simulink model "nn_12B"  (Simulink 10.0)
settings: Solver=ode45  StartTime=0  StopTime=100  RelTol=1e-3  EnableMultiTasking=on
values from neighbouring files (symbols this model uses):
  b1 = [-0.578256 -0.531049 0.449559 0.391358 0.277707 0.372638 -0.130073 0.423662 0.414256 -0.378106]    [nn_12B_data.mat]
  b2 = [-0.561938 -0.812212 -0.549473 -0.549797 -1.080223 0.652062 0.234581 1.306192 2.051893 -0.89138]    [nn_12B_data.mat]
  b3 = -0.01575    [nn_12B_data.mat]
  meaninp = [-0.014928 -0.08076]    [nn_12B_data.mat]
  meanout = -0.01416    [nn_12B_data.mat]
  oostdinp = [0.918012 0.847388]    [nn_12B_data.mat]
  stdevout = 0.183766    [nn_12B_data.mat]
  w1 = [-0.65101 1.000785 -0.225403 -1.250849 0.006928 0.402083 -0.27538 -0.375693 -0.343296 -0.963722 0.413488 0.166138 ... (20 elements, 2x10)]    [nn_12B_data.mat]
  w2 = [-0.059798 -0.128454 -0.107191 0.724165 -0.291639 -0.929753 -0.379182 0.996259 -0.416213 0.884865 -0.710416 -0.421403 ... (100 elements, 10x10)]    [nn_12B_data.mat]
  w3 = [-0.482061 0.739126 0.886125 1.875287 -0.959398 1.77256 -0.303801 0.909694 -0.681003 -0.930787]    [nn_12B_data.mat]
  xinmax = [1.885733 1.974943]    [nn_12B_data.mat]
  xinmin = [-1.969179 -1.999644]    [nn_12B_data.mat]
(part 1 of 2)
settings Model: Creator=niestma  LastModifiedBy=hbourbou
settings DataIOCC: LimitDataPoints=on
settings OptimizationCC: ExpressionDepthLimit=2147483647  LifeSpan=1  EfficientTunableParamExpr=on
settings DebuggingCC: StateNameClashWarn=warning
settings SFSimCC: MATLABDynamicMemAlloc=off
settings RTWCC: Description=Embedded Coder  SystemTargetFile=ert.tlc  TemplateMakefile=ert_default_tmf  GenerateReport=on  IncludeHyperlinkInReport=on  LaunchReport=on
settings CodeAppCC: IgnoreCustomStorageClasses=off  CustomSymbolStrType=$N$R$M  InternalIdentifier=Classic
settings ERTTargetCC: MultiwordLength=2048  GenerateSampleERTMain=on  ERTCustomFileTemplate=example_file_process.tlc  ConvertIfToSwitch=off  SuppressUnreachableDefaultCases=off
settings ConfigComp: CovExternalEMLEnable=off

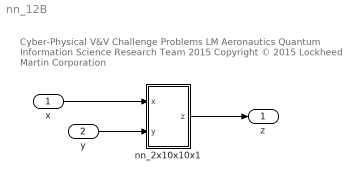
== system nn_12B ==
  note: Cyber-Physical V&V Challenge Problems
      | LM Aeronautics Quantum Information Science Research Team 2015
      | Copyright © 2015 Lockheed Martin Corporation
  x : Inport  OutDataTypeStr=double
  y : Inport  Port=2  OutDataTypeStr=double
  nn_2x10x10x1 : Subsystem
  z : Outport  VectorParamsAs1DForOutWhenUnconnected=off
  wires:
  nn_2x10x10x1/1(z) -> z/1
  x/1 -> nn_2x10x10x1/1(x)
  y/1 -> nn_2x10x10x1/2(y)

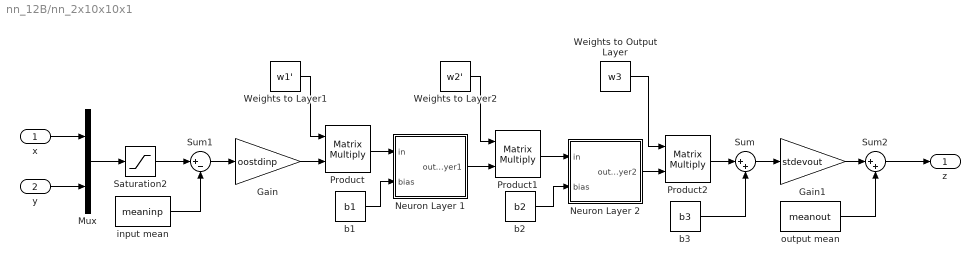
== system nn_12B/nn_2x10x10x1 ==
  x : Inport
  y : Inport  Port=2
  Gain : Gain  Gain=oostdinp
  Gain1 : Gain  Gain=stdevout
  Mux : Mux  Inputs=2
  Neuron Layer 1 : Subsystem
  Neuron Layer 2 : Subsystem
  Product : Product  Multiplication=Matrix(*)  RndMeth=Zero
  Product1 : Product  Multiplication=Matrix(*)  RndMeth=Zero
  Product2 : Product  Multiplication=Matrix(*)  RndMeth=Zero
  Saturation2 : Saturate  UpperLimit=xinmax  LowerLimit=xinmin
  Sum : Sum  Inputs=|++
  Sum1 : Sum  Inputs=|+-
  Sum2 : Sum  Inputs=|++
  Weights to Layer1 : Constant  Value=w1'  VectorParams1D=off
  Weights to Layer2 : Constant  Value=w2'  VectorParams1D=off
  Weights to Output Layer : Constant  Value=w3  VectorParams1D=off
  b1 : Constant  Value=b1
  b2 : Constant  Value=b2
  b3 : Constant  Value=b3
  input mean : Constant  Value=meaninp
  output mean : Constant  Value=meanout
  z : Outport  VectorParamsAs1DForOutWhenUnconnected=off
  wires:
  Product1/1 -> Neuron Layer 2/1(in)
  b2/1 -> Neuron Layer 2/2(bias)
  x/1 -> Mux/1
  b1/1 -> Neuron Layer 1/2(bias)
  b3/1 -> Sum/2
  y/1 -> Mux/2
  Weights to Layer1/1 -> Product/1
  Weights to Layer2/1 -> Product1/1
  Product/1 -> Neuron Layer 1/1(in)
  Neuron Layer 1/1(output layer1) -> Product1/2
  Weights to Output Layer/1 -> Product2/1
  Neuron Layer 2/1(output layer2) -> Product2/2
  Product2/1 -> Sum/1
  Mux/1 -> Saturation2/1
  Saturation2/1 -> Sum1/1
  input mean/1 -> Sum1/2
  Gain/1 -> Product/2
  Sum1/1 -> Gain/1
  Sum/1 -> Gain1/1
  Gain1/1 -> Sum2/1
  Sum2/1 -> z/1
  output mean/1 -> Sum2/2

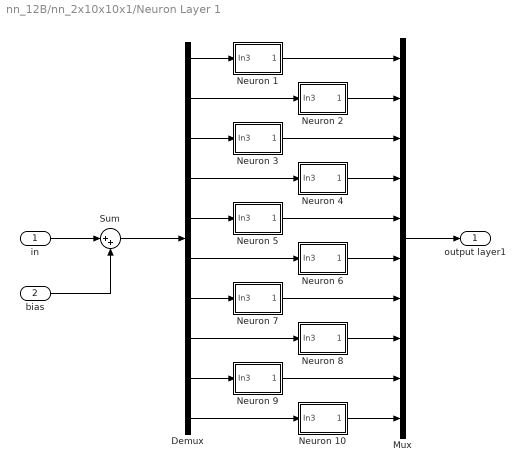
== system nn_12B/nn_2x10x10x1/Neuron Layer 1 ==
  in : Inport
  bias : Inport  Port=2
  Demux : Demux  Outputs=10
  Mux : Mux  Inputs=10
  Neuron 1 : Subsystem
  Neuron 10 : Subsystem
  Neuron 2 : Subsystem
  Neuron 3 : Subsystem
  Neuron 4 : Subsystem
  Neuron 5 : Subsystem
  Neuron 6 : Subsystem
  Neuron 7 : Subsystem
  Neuron 8 : Subsystem
  Neuron 9 : Subsystem
  Sum : Sum  Inputs=|++
  output layer1 : Outport  VectorParamsAs1DForOutWhenUnconnected=off
  wires:
  bias/1 -> Sum/2
  in/1 -> Sum/1
  Sum/1 -> Demux/1
  Demux/1 -> Neuron 1/1(In3)
  Neuron 1/1(Out1) -> Mux/1
  Mux/1 -> output layer1/1
  Neuron 2/1(Out1) -> Mux/2
  Demux/2 -> Neuron 2/1(In3)
  Demux/3 -> Neuron 3/1(In3)
  Neuron 3/1(Out1) -> Mux/3
  Demux/4 -> Neuron 4/1(In3)
  Neuron 4/1(Out1) -> Mux/4
  Demux/5 -> Neuron 5/1(In3)
  Neuron 5/1(Out1) -> Mux/5
  Demux/6 -> Neuron 6/1(In3)
  Demux/7 -> Neuron 7/1(In3)
  Neuron 7/1(Out1) -> Mux/7
  Demux/8 -> Neuron 8/1(In3)
  Neuron 6/1(Out1) -> Mux/6
  Neuron 8/1(Out1) -> Mux/8
  Demux/9 -> Neuron 9/1(In3)
  Neuron 9/1(Out1) -> Mux/9
  Demux/10 -> Neuron 10/1(In3)
  Neuron 10/1(Out1) -> Mux/10

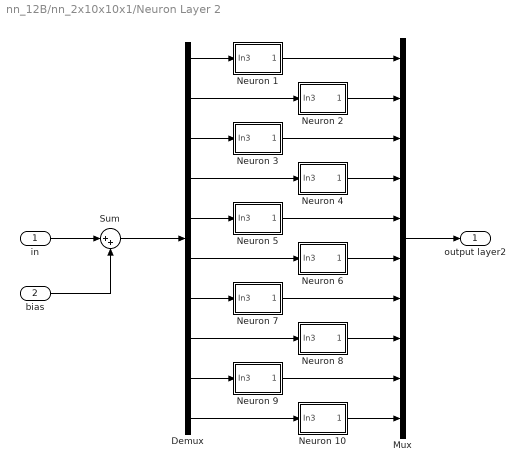
== system nn_12B/nn_2x10x10x1/Neuron Layer 2 ==
  in : Inport
  bias : Inport  Port=2
  Demux : Demux  Outputs=10
  Mux : Mux  Inputs=10
  Neuron 1 : Subsystem
  Neuron 10 : Subsystem
  Neuron 2 : Subsystem
  Neuron 3 : Subsystem
  Neuron 4 : Subsystem
  Neuron 5 : Subsystem
  Neuron 6 : Subsystem
  Neuron 7 : Subsystem
  Neuron 8 : Subsystem
  Neuron 9 : Subsystem
  Sum : Sum  Inputs=|++
  output layer2 : Outport  VectorParamsAs1DForOutWhenUnconnected=off
  wires:
  bias/1 -> Sum/2
  in/1 -> Sum/1
  Sum/1 -> Demux/1
  Demux/1 -> Neuron 1/1(In3)
  Neuron 1/1(Out1) -> Mux/1
  Mux/1 -> output layer2/1
  Neuron 2/1(Out1) -> Mux/2
  Demux/2 -> Neuron 2/1(In3)
  Demux/3 -> Neuron 3/1(In3)
  Neuron 3/1(Out1) -> Mux/3
  Demux/4 -> Neuron 4/1(In3)
  Neuron 4/1(Out1) -> Mux/4
  Demux/5 -> Neuron 5/1(In3)
  Neuron 5/1(Out1) -> Mux/5
  Demux/6 -> Neuron 6/1(In3)
  Demux/7 -> Neuron 7/1(In3)
  Neuron 7/1(Out1) -> Mux/7
  Demux/8 -> Neuron 8/1(In3)
  Neuron 6/1(Out1) -> Mux/6
  Neuron 8/1(Out1) -> Mux/8
  Demux/9 -> Neuron 9/1(In3)
  Neuron 9/1(Out1) -> Mux/9
  Demux/10 -> Neuron 10/1(In3)
  Neuron 10/1(Out1) -> Mux/10

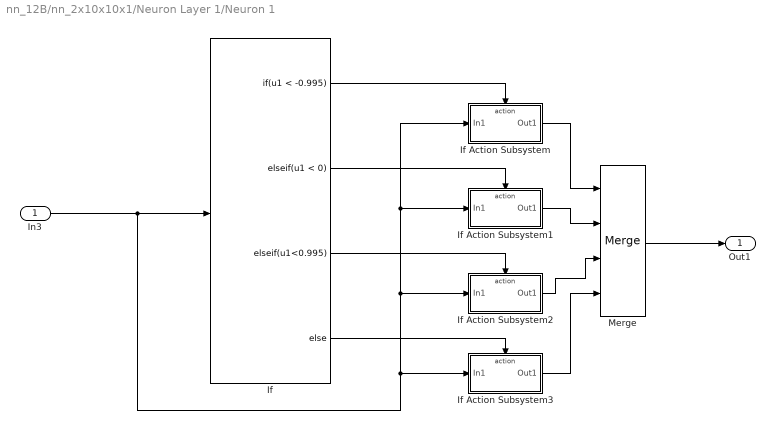
== system nn_12B/nn_2x10x10x1/Neuron Layer 1/Neuron 1 ==
  In3 : Inport
  If : If  IfExpression=u1 < -0.995  ElseIfExpressions=u1 < 0, u1<0.995
  If Action Subsystem : Subsystem  TreatAsAtomicUnit=on
  If Action Subsystem1 : Subsystem  TreatAsAtomicUnit=on
  If Action Subsystem2 : Subsystem  TreatAsAtomicUnit=on
  If Action Subsystem3 : Subsystem  TreatAsAtomicUnit=on
  Merge : Merge  Inputs=4
  Out1 : Outport  VectorParamsAs1DForOutWhenUnconnected=off
  wires:
  If/1 -> If Action Subsystem/Action
  If/2 -> If Action Subsystem1/Action
  If/3 -> If Action Subsystem2/Action
  If/4 -> If Action Subsystem3/Action
  If Action Subsystem/1(Out1) -> Merge/1
  If Action Subsystem3/1(Out1) -> Merge/4
  If Action Subsystem1/1(Out1) -> Merge/2
  If Action Subsystem2/1(Out1) -> Merge/3
  In3/1 -> If Action Subsystem3/1(In1), If Action Subsystem2/1(In1), If Action Subsystem1/1(In1), If Action Subsystem/1(In1), If/1
  Merge/1 -> Out1/1

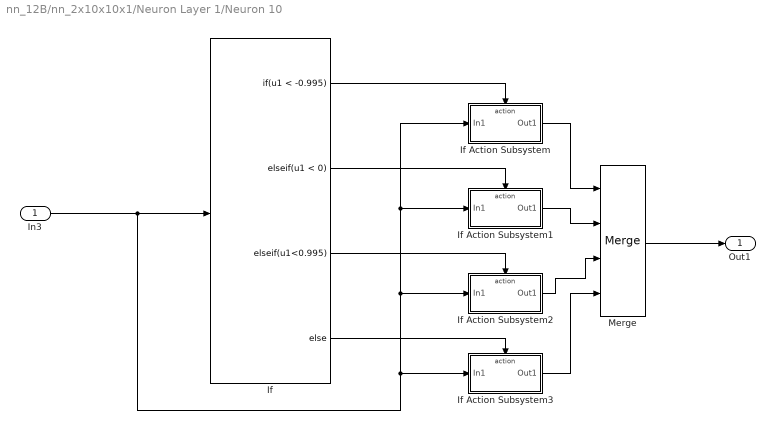
== system nn_12B/nn_2x10x10x1/Neuron Layer 1/Neuron 10 ==
  In3 : Inport
  If : If  IfExpression=u1 < -0.995  ElseIfExpressions=u1 < 0, u1<0.995
  If Action Subsystem : Subsystem  TreatAsAtomicUnit=on
  If Action Subsystem1 : Subsystem  TreatAsAtomicUnit=on
  If Action Subsystem2 : Subsystem  TreatAsAtomicUnit=on
  If Action Subsystem3 : Subsystem  TreatAsAtomicUnit=on
  Merge : Merge  Inputs=4
  Out1 : Outport  VectorParamsAs1DForOutWhenUnconnected=off
  wires:
  Merge/1 -> Out1/1
  In3/1 -> If/1, If Action Subsystem/1(In1), If Action Subsystem1/1(In1), If Action Subsystem2/1(In1), If Action Subsystem3/1(In1)
  If Action Subsystem2/1(Out1) -> Merge/3
  If Action Subsystem1/1(Out1) -> Merge/2
  If Action Subsystem3/1(Out1) -> Merge/4
  If Action Subsystem/1(Out1) -> Merge/1
  If/4 -> If Action Subsystem3/Action
  If/3 -> If Action Subsystem2/Action
  If/2 -> If Action Subsystem1/Action
  If/1 -> If Action Subsystem/Action

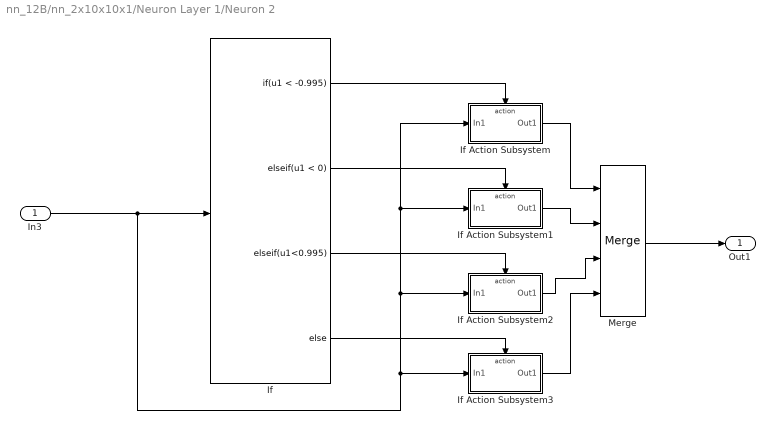
== system nn_12B/nn_2x10x10x1/Neuron Layer 1/Neuron 2 ==
  In3 : Inport
  If : If  IfExpression=u1 < -0.995  ElseIfExpressions=u1 < 0, u1<0.995
  If Action Subsystem : Subsystem  TreatAsAtomicUnit=on
  If Action Subsystem1 : Subsystem  TreatAsAtomicUnit=on
  If Action Subsystem2 : Subsystem  TreatAsAtomicUnit=on
  If Action Subsystem3 : Subsystem  TreatAsAtomicUnit=on
  Merge : Merge  Inputs=4
  Out1 : Outport  VectorParamsAs1DForOutWhenUnconnected=off
  wires:
  Merge/1 -> Out1/1
  In3/1 -> If/1, If Action Subsystem/1(In1), If Action Subsystem1/1(In1), If Action Subsystem2/1(In1), If Action Subsystem3/1(In1)
  If Action Subsystem2/1(Out1) -> Merge/3
  If Action Subsystem1/1(Out1) -> Merge/2
  If Action Subsystem3/1(Out1) -> Merge/4
  If Action Subsystem/1(Out1) -> Merge/1
  If/4 -> If Action Subsystem3/Action
  If/3 -> If Action Subsystem2/Action
  If/2 -> If Action Subsystem1/Action
  If/1 -> If Action Subsystem/Action

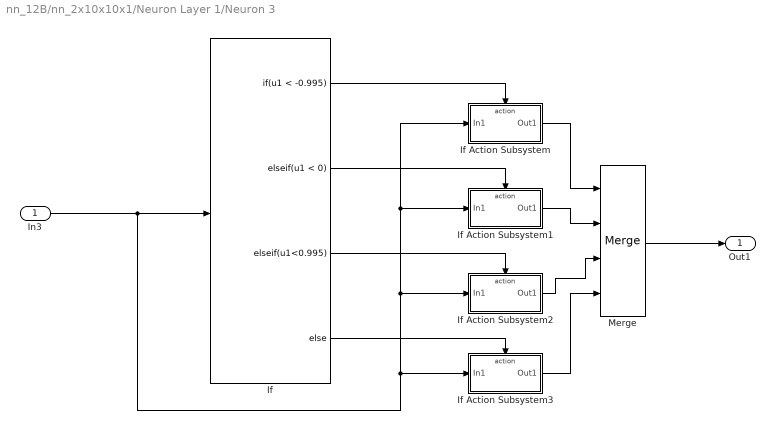
== system nn_12B/nn_2x10x10x1/Neuron Layer 1/Neuron 3 ==
  In3 : Inport
  If : If  IfExpression=u1 < -0.995  ElseIfExpressions=u1 < 0, u1<0.995
  If Action Subsystem : Subsystem  TreatAsAtomicUnit=on
  If Action Subsystem1 : Subsystem  TreatAsAtomicUnit=on
  If Action Subsystem2 : Subsystem  TreatAsAtomicUnit=on
  If Action Subsystem3 : Subsystem  TreatAsAtomicUnit=on
  Merge : Merge  Inputs=4
  Out1 : Outport  VectorParamsAs1DForOutWhenUnconnected=off
  wires:
  If/1 -> If Action Subsystem/Action
  If/2 -> If Action Subsystem1/Action
  If/3 -> If Action Subsystem2/Action
  If/4 -> If Action Subsystem3/Action
  If Action Subsystem/1(Out1) -> Merge/1
  If Action Subsystem3/1(Out1) -> Merge/4
  If Action Subsystem1/1(Out1) -> Merge/2
  If Action Subsystem2/1(Out1) -> Merge/3
  In3/1 -> If Action Subsystem3/1(In1), If Action Subsystem2/1(In1), If Action Subsystem1/1(In1), If Action Subsystem/1(In1), If/1
  Merge/1 -> Out1/1

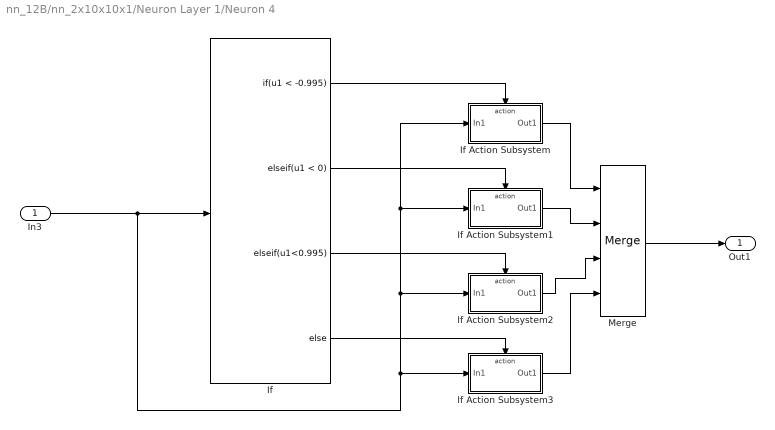
== system nn_12B/nn_2x10x10x1/Neuron Layer 1/Neuron 4 ==
  In3 : Inport
  If : If  IfExpression=u1 < -0.995  ElseIfExpressions=u1 < 0, u1<0.995
  If Action Subsystem : Subsystem  TreatAsAtomicUnit=on
  If Action Subsystem1 : Subsystem  TreatAsAtomicUnit=on
  If Action Subsystem2 : Subsystem  TreatAsAtomicUnit=on
  If Action Subsystem3 : Subsystem  TreatAsAtomicUnit=on
  Merge : Merge  Inputs=4
  Out1 : Outport  VectorParamsAs1DForOutWhenUnconnected=off
  wires:
  If/1 -> If Action Subsystem/Action
  If/2 -> If Action Subsystem1/Action
  If/3 -> If Action Subsystem2/Action
  If/4 -> If Action Subsystem3/Action
  If Action Subsystem/1(Out1) -> Merge/1
  If Action Subsystem3/1(Out1) -> Merge/4
  If Action Subsystem1/1(Out1) -> Merge/2
  If Action Subsystem2/1(Out1) -> Merge/3
  In3/1 -> If Action Subsystem3/1(In1), If Action Subsystem2/1(In1), If Action Subsystem1/1(In1), If Action Subsystem/1(In1), If/1
  Merge/1 -> Out1/1

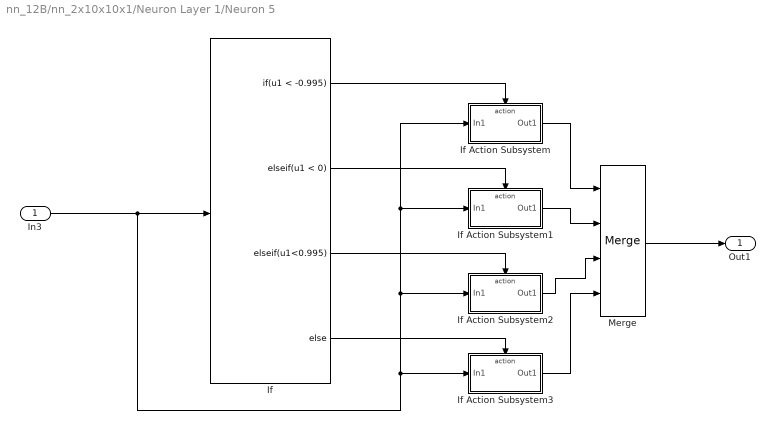
== system nn_12B/nn_2x10x10x1/Neuron Layer 1/Neuron 5 ==
  In3 : Inport
  If : If  IfExpression=u1 < -0.995  ElseIfExpressions=u1 < 0, u1<0.995
  If Action Subsystem : Subsystem  TreatAsAtomicUnit=on
  If Action Subsystem1 : Subsystem  TreatAsAtomicUnit=on
  If Action Subsystem2 : Subsystem  TreatAsAtomicUnit=on
  If Action Subsystem3 : Subsystem  TreatAsAtomicUnit=on
  Merge : Merge  Inputs=4
  Out1 : Outport  VectorParamsAs1DForOutWhenUnconnected=off
  wires:
  If/1 -> If Action Subsystem/Action
  If/2 -> If Action Subsystem1/Action
  If/3 -> If Action Subsystem2/Action
  If/4 -> If Action Subsystem3/Action
  If Action Subsystem/1(Out1) -> Merge/1
  If Action Subsystem3/1(Out1) -> Merge/4
  If Action Subsystem1/1(Out1) -> Merge/2
  If Action Subsystem2/1(Out1) -> Merge/3
  In3/1 -> If Action Subsystem3/1(In1), If Action Subsystem2/1(In1), If Action Subsystem1/1(In1), If Action Subsystem/1(In1), If/1
  Merge/1 -> Out1/1

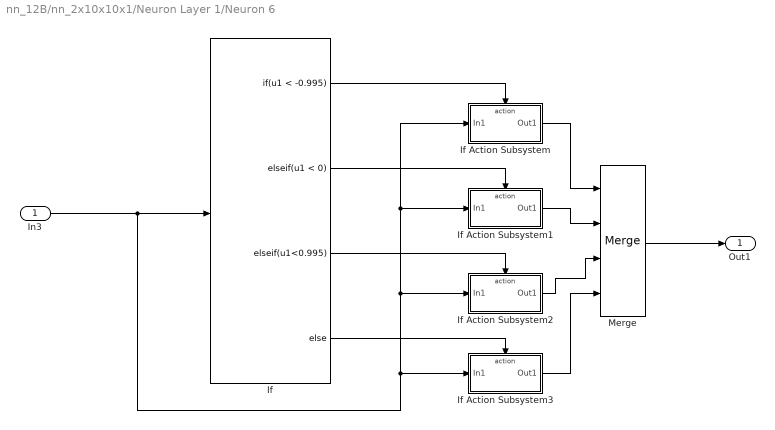
== system nn_12B/nn_2x10x10x1/Neuron Layer 1/Neuron 6 ==
  In3 : Inport
  If : If  IfExpression=u1 < -0.995  ElseIfExpressions=u1 < 0, u1<0.995
  If Action Subsystem : Subsystem  TreatAsAtomicUnit=on
  If Action Subsystem1 : Subsystem  TreatAsAtomicUnit=on
  If Action Subsystem2 : Subsystem  TreatAsAtomicUnit=on
  If Action Subsystem3 : Subsystem  TreatAsAtomicUnit=on
  Merge : Merge  Inputs=4
  Out1 : Outport  VectorParamsAs1DForOutWhenUnconnected=off
  wires:
  Merge/1 -> Out1/1
  In3/1 -> If/1, If Action Subsystem/1(In1), If Action Subsystem1/1(In1), If Action Subsystem2/1(In1), If Action Subsystem3/1(In1)
  If Action Subsystem2/1(Out1) -> Merge/3
  If Action Subsystem1/1(Out1) -> Merge/2
  If Action Subsystem3/1(Out1) -> Merge/4
  If Action Subsystem/1(Out1) -> Merge/1
  If/4 -> If Action Subsystem3/Action
  If/3 -> If Action Subsystem2/Action
  If/2 -> If Action Subsystem1/Action
  If/1 -> If Action Subsystem/Action

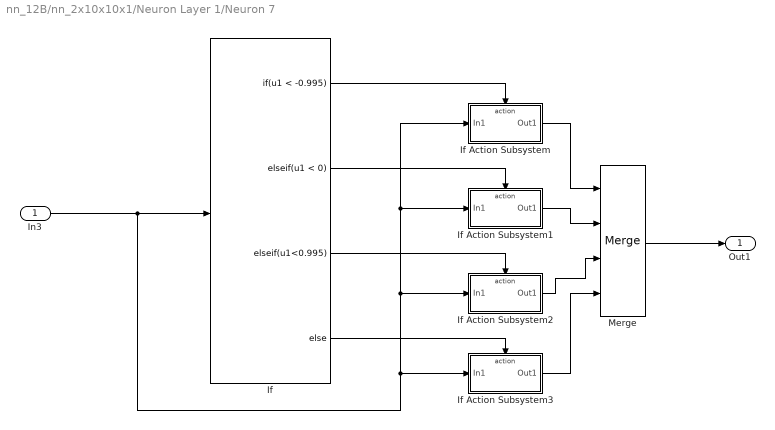
== system nn_12B/nn_2x10x10x1/Neuron Layer 1/Neuron 7 ==
  In3 : Inport
  If : If  IfExpression=u1 < -0.995  ElseIfExpressions=u1 < 0, u1<0.995
  If Action Subsystem : Subsystem  TreatAsAtomicUnit=on
  If Action Subsystem1 : Subsystem  TreatAsAtomicUnit=on
  If Action Subsystem2 : Subsystem  TreatAsAtomicUnit=on
  If Action Subsystem3 : Subsystem  TreatAsAtomicUnit=on
  Merge : Merge  Inputs=4
  Out1 : Outport  VectorParamsAs1DForOutWhenUnconnected=off
  wires:
  If/1 -> If Action Subsystem/Action
  If/2 -> If Action Subsystem1/Action
  If/3 -> If Action Subsystem2/Action
  If/4 -> If Action Subsystem3/Action
  If Action Subsystem/1(Out1) -> Merge/1
  If Action Subsystem3/1(Out1) -> Merge/4
  If Action Subsystem1/1(Out1) -> Merge/2
  If Action Subsystem2/1(Out1) -> Merge/3
  In3/1 -> If Action Subsystem3/1(In1), If Action Subsystem2/1(In1), If Action Subsystem1/1(In1), If Action Subsystem/1(In1), If/1
  Merge/1 -> Out1/1

== system nn_12B/nn_2x10x10x1/Neuron Layer 1/Neuron 8 ==
  In3 : Inport
  If : If  IfExpression=u1 < -0.995  ElseIfExpressions=u1 < 0, u1<0.995
  If Action Subsystem : Subsystem  TreatAsAtomicUnit=on
  If Action Subsystem1 : Subsystem  TreatAsAtomicUnit=on
  If Action Subsystem2 : Subsystem  TreatAsAtomicUnit=on
  If Action Subsystem3 : Subsystem  TreatAsAtomicUnit=on
  Merge : Merge  Inputs=4
  Out1 : Outport  VectorParamsAs1DForOutWhenUnconnected=off
  wires:
  If/1 -> If Action Subsystem/Action
  If/2 -> If Action Subsystem1/Action
  If/3 -> If Action Subsystem2/Action
  If/4 -> If Action Subsystem3/Action
  If Action Subsystem/1(Out1) -> Merge/1
  If Action Subsystem3/1(Out1) -> Merge/4
  If Action Subsystem1/1(Out1) -> Merge/2
  If Action Subsystem2/1(Out1) -> Merge/3
  In3/1 -> If Action Subsystem3/1(In1), If Action Subsystem2/1(In1), If Action Subsystem1/1(In1), If Action Subsystem/1(In1), If/1
  Merge/1 -> Out1/1

== system nn_12B/nn_2x10x10x1/Neuron Layer 1/Neuron 9 ==
  In3 : Inport
  If : If  IfExpression=u1 < -0.995  ElseIfExpressions=u1 < 0, u1<0.995
  If Action Subsystem : Subsystem  TreatAsAtomicUnit=on
  If Action Subsystem1 : Subsystem  TreatAsAtomicUnit=on
  If Action Subsystem2 : Subsystem  TreatAsAtomicUnit=on
  If Action Subsystem3 : Subsystem  TreatAsAtomicUnit=on
  Merge : Merge  Inputs=4
  Out1 : Outport  VectorParamsAs1DForOutWhenUnconnected=off
  wires:
  If/1 -> If Action Subsystem/Action
  If/2 -> If Action Subsystem1/Action
  If/3 -> If Action Subsystem2/Action
  If/4 -> If Action Subsystem3/Action
  If Action Subsystem/1(Out1) -> Merge/1
  If Action Subsystem3/1(Out1) -> Merge/4
  If Action Subsystem1/1(Out1) -> Merge/2
  If Action Subsystem2/1(Out1) -> Merge/3
  In3/1 -> If Action Subsystem3/1(In1), If Action Subsystem2/1(In1), If Action Subsystem1/1(In1), If Action Subsystem/1(In1), If/1
  Merge/1 -> Out1/1

== system nn_12B/nn_2x10x10x1/Neuron Layer 2/Neuron 1 ==
  In3 : Inport
  If : If  IfExpression=u1 < -0.995  ElseIfExpressions=u1 < 0, u1<0.995
  If Action Subsystem : Subsystem  TreatAsAtomicUnit=on
  If Action Subsystem1 : Subsystem  TreatAsAtomicUnit=on
  If Action Subsystem2 : Subsystem  TreatAsAtomicUnit=on
  If Action Subsystem3 : Subsystem  TreatAsAtomicUnit=on
  Merge : Merge  Inputs=4
  Out1 : Outport  VectorParamsAs1DForOutWhenUnconnected=off
  wires:
  If/1 -> If Action Subsystem/Action
  If/2 -> If Action Subsystem1/Action
  If/3 -> If Action Subsystem2/Action
  If/4 -> If Action Subsystem3/Action
  If Action Subsystem/1(Out1) -> Merge/1
  If Action Subsystem3/1(Out1) -> Merge/4
  If Action Subsystem1/1(Out1) -> Merge/2
  If Action Subsystem2/1(Out1) -> Merge/3
  In3/1 -> If Action Subsystem3/1(In1), If Action Subsystem2/1(In1), If Action Subsystem1/1(In1), If Action Subsystem/1(In1), If/1
  Merge/1 -> Out1/1

== system nn_12B/nn_2x10x10x1/Neuron Layer 2/Neuron 10 ==
  In3 : Inport
  If : If  IfExpression=u1 < -0.995  ElseIfExpressions=u1 < 0, u1<0.995
  If Action Subsystem : Subsystem  TreatAsAtomicUnit=on
  If Action Subsystem1 : Subsystem  TreatAsAtomicUnit=on
  If Action Subsystem2 : Subsystem  TreatAsAtomicUnit=on
  If Action Subsystem3 : Subsystem  TreatAsAtomicUnit=on
  Merge : Merge  Inputs=4
  Out1 : Outport  VectorParamsAs1DForOutWhenUnconnected=off
  wires:
  Merge/1 -> Out1/1
  In3/1 -> If/1, If Action Subsystem/1(In1), If Action Subsystem1/1(In1), If Action Subsystem2/1(In1), If Action Subsystem3/1(In1)
  If Action Subsystem2/1(Out1) -> Merge/3
  If Action Subsystem1/1(Out1) -> Merge/2
  If Action Subsystem3/1(Out1) -> Merge/4
  If Action Subsystem/1(Out1) -> Merge/1
  If/4 -> If Action Subsystem3/Action
  If/3 -> If Action Subsystem2/Action
  If/2 -> If Action Subsystem1/Action
  If/1 -> If Action Subsystem/Action

== system nn_12B/nn_2x10x10x1/Neuron Layer 2/Neuron 2 ==
  In3 : Inport
  If : If  IfExpression=u1 < -0.995  ElseIfExpressions=u1 < 0, u1<0.995
  If Action Subsystem : Subsystem  TreatAsAtomicUnit=on
  If Action Subsystem1 : Subsystem  TreatAsAtomicUnit=on
  If Action Subsystem2 : Subsystem  TreatAsAtomicUnit=on
  If Action Subsystem3 : Subsystem  TreatAsAtomicUnit=on
  Merge : Merge  Inputs=4
  Out1 : Outport  VectorParamsAs1DForOutWhenUnconnected=off
  wires:
  Merge/1 -> Out1/1
  In3/1 -> If/1, If Action Subsystem/1(In1), If Action Subsystem1/1(In1), If Action Subsystem2/1(In1), If Action Subsystem3/1(In1)
  If Action Subsystem2/1(Out1) -> Merge/3
  If Action Subsystem1/1(Out1) -> Merge/2
  If Action Subsystem3/1(Out1) -> Merge/4
  If Action Subsystem/1(Out1) -> Merge/1
  If/4 -> If Action Subsystem3/Action
  If/3 -> If Action Subsystem2/Action
  If/2 -> If Action Subsystem1/Action
  If/1 -> If Action Subsystem/Action

== system nn_12B/nn_2x10x10x1/Neuron Layer 2/Neuron 3 ==
  In3 : Inport
  If : If  IfExpression=u1 < -0.995  ElseIfExpressions=u1 < 0, u1<0.995
  If Action Subsystem : Subsystem  TreatAsAtomicUnit=on
  If Action Subsystem1 : Subsystem  TreatAsAtomicUnit=on
  If Action Subsystem2 : Subsystem  TreatAsAtomicUnit=on
  If Action Subsystem3 : Subsystem  TreatAsAtomicUnit=on
  Merge : Merge  Inputs=4
  Out1 : Outport  VectorParamsAs1DForOutWhenUnconnected=off
  wires:
  If/1 -> If Action Subsystem/Action
  If/2 -> If Action Subsystem1/Action
  If/3 -> If Action Subsystem2/Action
  If/4 -> If Action Subsystem3/Action
  If Action Subsystem/1(Out1) -> Merge/1
  If Action Subsystem3/1(Out1) -> Merge/4
  If Action Subsystem1/1(Out1) -> Merge/2
  If Action Subsystem2/1(Out1) -> Merge/3
  In3/1 -> If Action Subsystem3/1(In1), If Action Subsystem2/1(In1), If Action Subsystem1/1(In1), If Action Subsystem/1(In1), If/1
  Merge/1 -> Out1/1

== system nn_12B/nn_2x10x10x1/Neuron Layer 2/Neuron 4 ==
  In3 : Inport
  If : If  IfExpression=u1 < -0.995  ElseIfExpressions=u1 < 0, u1<0.995
  If Action Subsystem : Subsystem  TreatAsAtomicUnit=on
  If Action Subsystem1 : Subsystem  TreatAsAtomicUnit=on
  If Action Subsystem2 : Subsystem  TreatAsAtomicUnit=on
  If Action Subsystem3 : Subsystem  TreatAsAtomicUnit=on
  Merge : Merge  Inputs=4
  Out1 : Outport  VectorParamsAs1DForOutWhenUnconnected=off
  wires:
  If/1 -> If Action Subsystem/Action
  If/2 -> If Action Subsystem1/Action
  If/3 -> If Action Subsystem2/Action
  If/4 -> If Action Subsystem3/Action
  If Action Subsystem/1(Out1) -> Merge/1
  If Action Subsystem3/1(Out1) -> Merge/4
  If Action Subsystem1/1(Out1) -> Merge/2
  If Action Subsystem2/1(Out1) -> Merge/3
  In3/1 -> If Action Subsystem3/1(In1), If Action Subsystem2/1(In1), If Action Subsystem1/1(In1), If Action Subsystem/1(In1), If/1
  Merge/1 -> Out1/1

== system nn_12B/nn_2x10x10x1/Neuron Layer 2/Neuron 5 ==
  In3 : Inport
  If : If  IfExpression=u1 < -0.995  ElseIfExpressions=u1 < 0, u1<0.995
  If Action Subsystem : Subsystem  TreatAsAtomicUnit=on
  If Action Subsystem1 : Subsystem  TreatAsAtomicUnit=on
  If Action Subsystem2 : Subsystem  TreatAsAtomicUnit=on
  If Action Subsystem3 : Subsystem  TreatAsAtomicUnit=on
  Merge : Merge  Inputs=4
  Out1 : Outport  VectorParamsAs1DForOutWhenUnconnected=off
  wires:
  If/1 -> If Action Subsystem/Action
  If/2 -> If Action Subsystem1/Action
  If/3 -> If Action Subsystem2/Action
  If/4 -> If Action Subsystem3/Action
  If Action Subsystem/1(Out1) -> Merge/1
  If Action Subsystem3/1(Out1) -> Merge/4
  If Action Subsystem1/1(Out1) -> Merge/2
  If Action Subsystem2/1(Out1) -> Merge/3
  In3/1 -> If Action Subsystem3/1(In1), If Action Subsystem2/1(In1), If Action Subsystem1/1(In1), If Action Subsystem/1(In1), If/1
  Merge/1 -> Out1/1

== system nn_12B/nn_2x10x10x1/Neuron Layer 2/Neuron 6 ==
  In3 : Inport
  If : If  IfExpression=u1 < -0.995  ElseIfExpressions=u1 < 0, u1<0.995
  If Action Subsystem : Subsystem  TreatAsAtomicUnit=on
  If Action Subsystem1 : Subsystem  TreatAsAtomicUnit=on
  If Action Subsystem2 : Subsystem  TreatAsAtomicUnit=on
  If Action Subsystem3 : Subsystem  TreatAsAtomicUnit=on
  Merge : Merge  Inputs=4
  Out1 : Outport  VectorParamsAs1DForOutWhenUnconnected=off
  wires:
  Merge/1 -> Out1/1
  In3/1 -> If/1, If Action Subsystem/1(In1), If Action Subsystem1/1(In1), If Action Subsystem2/1(In1), If Action Subsystem3/1(In1)
  If Action Subsystem2/1(Out1) -> Merge/3
  If Action Subsystem1/1(Out1) -> Merge/2
  If Action Subsystem3/1(Out1) -> Merge/4
  If Action Subsystem/1(Out1) -> Merge/1
  If/4 -> If Action Subsystem3/Action
  If/3 -> If Action Subsystem2/Action
  If/2 -> If Action Subsystem1/Action
  If/1 -> If Action Subsystem/Action

== system nn_12B/nn_2x10x10x1/Neuron Layer 2/Neuron 7 ==
  In3 : Inport
  If : If  IfExpression=u1 < -0.995  ElseIfExpressions=u1 < 0, u1<0.995
  If Action Subsystem : Subsystem  TreatAsAtomicUnit=on
  If Action Subsystem1 : Subsystem  TreatAsAtomicUnit=on
  If Action Subsystem2 : Subsystem  TreatAsAtomicUnit=on
  If Action Subsystem3 : Subsystem  TreatAsAtomicUnit=on
  Merge : Merge  Inputs=4
  Out1 : Outport  VectorParamsAs1DForOutWhenUnconnected=off
  wires:
  If/1 -> If Action Subsystem/Action
  If/2 -> If Action Subsystem1/Action
  If/3 -> If Action Subsystem2/Action
  If/4 -> If Action Subsystem3/Action
  If Action Subsystem/1(Out1) -> Merge/1
  If Action Subsystem3/1(Out1) -> Merge/4
  If Action Subsystem1/1(Out1) -> Merge/2
  If Action Subsystem2/1(Out1) -> Merge/3
  In3/1 -> If Action Subsystem3/1(In1), If Action Subsystem2/1(In1), If Action Subsystem1/1(In1), If Action Subsystem/1(In1), If/1
  Merge/1 -> Out1/1

== system nn_12B/nn_2x10x10x1/Neuron Layer 2/Neuron 8 ==
  In3 : Inport
  If : If  IfExpression=u1 < -0.995  ElseIfExpressions=u1 < 0, u1<0.995
  If Action Subsystem : Subsystem  TreatAsAtomicUnit=on
  If Action Subsystem1 : Subsystem  TreatAsAtomicUnit=on
  If Action Subsystem2 : Subsystem  TreatAsAtomicUnit=on
  If Action Subsystem3 : Subsystem  TreatAsAtomicUnit=on
  Merge : Merge  Inputs=4
  Out1 : Outport  VectorParamsAs1DForOutWhenUnconnected=off
  wires:
  If/1 -> If Action Subsystem/Action
  If/2 -> If Action Subsystem1/Action
  If/3 -> If Action Subsystem2/Action
  If/4 -> If Action Subsystem3/Action
  If Action Subsystem/1(Out1) -> Merge/1
  If Action Subsystem3/1(Out1) -> Merge/4
  If Action Subsystem1/1(Out1) -> Merge/2
  If Action Subsystem2/1(Out1) -> Merge/3
  In3/1 -> If Action Subsystem3/1(In1), If Action Subsystem2/1(In1), If Action Subsystem1/1(In1), If Action Subsystem/1(In1), If/1
  Merge/1 -> Out1/1

== system nn_12B/nn_2x10x10x1/Neuron Layer 2/Neuron 9 ==
  In3 : Inport
  If : If  IfExpression=u1 < -0.995  ElseIfExpressions=u1 < 0, u1<0.995
  If Action Subsystem : Subsystem  TreatAsAtomicUnit=on
  If Action Subsystem1 : Subsystem  TreatAsAtomicUnit=on
  If Action Subsystem2 : Subsystem  TreatAsAtomicUnit=on
  If Action Subsystem3 : Subsystem  TreatAsAtomicUnit=on
  Merge : Merge  Inputs=4
  Out1 : Outport  VectorParamsAs1DForOutWhenUnconnected=off
  wires:
  If/1 -> If Action Subsystem/Action
  If/2 -> If Action Subsystem1/Action
  If/3 -> If Action Subsystem2/Action
  If/4 -> If Action Subsystem3/Action
  If Action Subsystem/1(Out1) -> Merge/1
  If Action Subsystem3/1(Out1) -> Merge/4
  If Action Subsystem1/1(Out1) -> Merge/2
  If Action Subsystem2/1(Out1) -> Merge/3
  In3/1 -> If Action Subsystem3/1(In1), If Action Subsystem2/1(In1), If Action Subsystem1/1(In1), If Action Subsystem/1(In1), If/1
  Merge/1 -> Out1/1

== system nn_12B/nn_2x10x10x1/Neuron Layer 1/Neuron 1/If Action Subsystem ==
  In1 : Inport
  Action Port : ActionPort  ActionPortLabel=if { }
  Sum : Sum  Inputs=|+-
  bias1 : Constant  Value=0.990025
  weight1 : Gain  Gain=0.01
  Out1 : Outport  VectorParamsAs1DForOutWhenUnconnected=off
  wires:
  bias1/1 -> Sum/2
  weight1/1 -> Sum/1
  In1/1 -> weight1/1
  Sum/1 -> Out1/1

== system nn_12B/nn_2x10x10x1/Neuron Layer 1/Neuron 1/If Action Subsystem1 ==
  In1 : Inport
  Action Port : ActionPort  ActionPortLabel=elseif { }
  Product1 : Product  RndMeth=Zero
  Sum3 : Sum  Inputs=|++
  bias4 : Constant  Value=2
  Out1 : Outport  VectorParamsAs1DForOutWhenUnconnected=off
  wires:
  In1/1 -> Product1/1, Sum3/1
  bias4/1 -> Sum3/2
  Sum3/1 -> Product1/2
  Product1/1 -> Out1/1

== system nn_12B/nn_2x10x10x1/Neuron Layer 1/Neuron 1/If Action Subsystem2 ==
  In1 : Inport
  Action Port : ActionPort  ActionPortLabel=elseif { }
  Product1 : Product  RndMeth=Zero
  Sum3 : Sum  Inputs=|-+
  bias4 : Constant  Value=2
  Out1 : Outport  VectorParamsAs1DForOutWhenUnconnected=off
  wires:
  Product1/1 -> Out1/1
  Sum3/1 -> Product1/2
  bias4/1 -> Sum3/2
  In1/1 -> Sum3/1, Product1/1

== system nn_12B/nn_2x10x10x1/Neuron Layer 1/Neuron 1/If Action Subsystem3 ==
  In1 : Inport
  Action Port : ActionPort  ActionPortLabel=else { }
  Sum : Sum  Inputs=|++
  bias1 : Constant  Value=0.990025
  weight1 : Gain  Gain=0.01
  Out1 : Outport  VectorParamsAs1DForOutWhenUnconnected=off
  wires:
  bias1/1 -> Sum/2
  weight1/1 -> Sum/1
  In1/1 -> weight1/1
  Sum/1 -> Out1/1

== system nn_12B/nn_2x10x10x1/Neuron Layer 1/Neuron 10/If Action Subsystem ==
  In1 : Inport
  Action Port : ActionPort  ActionPortLabel=if { }
  Sum : Sum  Inputs=|+-
  bias1 : Constant  Value=0.990025
  weight1 : Gain  Gain=0.01
  Out1 : Outport  VectorParamsAs1DForOutWhenUnconnected=off
  wires:
  Sum/1 -> Out1/1
  In1/1 -> weight1/1
  weight1/1 -> Sum/1
  bias1/1 -> Sum/2

== system nn_12B/nn_2x10x10x1/Neuron Layer 1/Neuron 10/If Action Subsystem1 ==
  In1 : Inport
  Action Port : ActionPort  ActionPortLabel=elseif { }
  Product1 : Product  RndMeth=Zero
  Sum3 : Sum  Inputs=|++
  bias4 : Constant  Value=2
  Out1 : Outport  VectorParamsAs1DForOutWhenUnconnected=off
  wires:
  Product1/1 -> Out1/1
  Sum3/1 -> Product1/2
  bias4/1 -> Sum3/2
  In1/1 -> Sum3/1, Product1/1

== system nn_12B/nn_2x10x10x1/Neuron Layer 1/Neuron 10/If Action Subsystem2 ==
  In1 : Inport
  Action Port : ActionPort  ActionPortLabel=elseif { }
  Product1 : Product  RndMeth=Zero
  Sum3 : Sum  Inputs=|-+
  bias4 : Constant  Value=2
  Out1 : Outport  VectorParamsAs1DForOutWhenUnconnected=off
  wires:
  In1/1 -> Product1/1, Sum3/1
  bias4/1 -> Sum3/2
  Sum3/1 -> Product1/2
  Product1/1 -> Out1/1

== system nn_12B/nn_2x10x10x1/Neuron Layer 1/Neuron 10/If Action Subsystem3 ==
  In1 : Inport
  Action Port : ActionPort  ActionPortLabel=else { }
  Sum : Sum  Inputs=|++
  bias1 : Constant  Value=0.990025
  weight1 : Gain  Gain=0.01
  Out1 : Outport  VectorParamsAs1DForOutWhenUnconnected=off
  wires:
  Sum/1 -> Out1/1
  In1/1 -> weight1/1
  weight1/1 -> Sum/1
  bias1/1 -> Sum/2

== system nn_12B/nn_2x10x10x1/Neuron Layer 1/Neuron 2/If Action Subsystem ==
  In1 : Inport
  Action Port : ActionPort  ActionPortLabel=if { }
  Sum : Sum  Inputs=|+-
  bias1 : Constant  Value=0.990025
  weight1 : Gain  Gain=0.01
  Out1 : Outport  VectorParamsAs1DForOutWhenUnconnected=off
  wires:
  Sum/1 -> Out1/1
  In1/1 -> weight1/1
  weight1/1 -> Sum/1
  bias1/1 -> Sum/2

== system nn_12B/nn_2x10x10x1/Neuron Layer 1/Neuron 2/If Action Subsystem1 ==
  In1 : Inport
  Action Port : ActionPort  ActionPortLabel=elseif { }
  Product1 : Product  RndMeth=Zero
  Sum3 : Sum  Inputs=|++
  bias4 : Constant  Value=2
  Out1 : Outport  VectorParamsAs1DForOutWhenUnconnected=off
  wires:
  Product1/1 -> Out1/1
  Sum3/1 -> Product1/2
  bias4/1 -> Sum3/2
  In1/1 -> Sum3/1, Product1/1

== system nn_12B/nn_2x10x10x1/Neuron Layer 1/Neuron 2/If Action Subsystem2 ==
  In1 : Inport
  Action Port : ActionPort  ActionPortLabel=elseif { }
  Product1 : Product  RndMeth=Zero
  Sum3 : Sum  Inputs=|-+
  bias4 : Constant  Value=2
  Out1 : Outport  VectorParamsAs1DForOutWhenUnconnected=off
  wires:
  In1/1 -> Product1/1, Sum3/1
  bias4/1 -> Sum3/2
  Sum3/1 -> Product1/2
  Product1/1 -> Out1/1

== system nn_12B/nn_2x10x10x1/Neuron Layer 1/Neuron 2/If Action Subsystem3 ==
  In1 : Inport
  Action Port : ActionPort  ActionPortLabel=else { }
  Sum : Sum  Inputs=|++
  bias1 : Constant  Value=0.990025
  weight1 : Gain  Gain=0.01
  Out1 : Outport  VectorParamsAs1DForOutWhenUnconnected=off
  wires:
  Sum/1 -> Out1/1
  In1/1 -> weight1/1
  weight1/1 -> Sum/1
  bias1/1 -> Sum/2

== system nn_12B/nn_2x10x10x1/Neuron Layer 1/Neuron 3/If Action Subsystem ==
  In1 : Inport
  Action Port : ActionPort  ActionPortLabel=if { }
  Sum : Sum  Inputs=|+-
  bias1 : Constant  Value=0.990025
  weight1 : Gain  Gain=0.01
  Out1 : Outport  VectorParamsAs1DForOutWhenUnconnected=off
  wires:
  bias1/1 -> Sum/2
  weight1/1 -> Sum/1
  In1/1 -> weight1/1
  Sum/1 -> Out1/1

== system nn_12B/nn_2x10x10x1/Neuron Layer 1/Neuron 3/If Action Subsystem1 ==
  In1 : Inport
  Action Port : ActionPort  ActionPortLabel=elseif { }
  Product1 : Product  RndMeth=Zero
  Sum3 : Sum  Inputs=|++
  bias4 : Constant  Value=2
  Out1 : Outport  VectorParamsAs1DForOutWhenUnconnected=off
  wires:
  In1/1 -> Product1/1, Sum3/1
  bias4/1 -> Sum3/2
  Sum3/1 -> Product1/2
  Product1/1 -> Out1/1

== system nn_12B/nn_2x10x10x1/Neuron Layer 1/Neuron 3/If Action Subsystem2 ==
  In1 : Inport
  Action Port : ActionPort  ActionPortLabel=elseif { }
  Product1 : Product  RndMeth=Zero
  Sum3 : Sum  Inputs=|-+
  bias4 : Constant  Value=2
  Out1 : Outport  VectorParamsAs1DForOutWhenUnconnected=off
  wires:
  Product1/1 -> Out1/1
  Sum3/1 -> Product1/2
  bias4/1 -> Sum3/2
  In1/1 -> Sum3/1, Product1/1

== system nn_12B/nn_2x10x10x1/Neuron Layer 1/Neuron 3/If Action Subsystem3 ==
  In1 : Inport
  Action Port : ActionPort  ActionPortLabel=else { }
  Sum : Sum  Inputs=|++
  bias1 : Constant  Value=0.990025
  weight1 : Gain  Gain=0.01
  Out1 : Outport  VectorParamsAs1DForOutWhenUnconnected=off
  wires:
  bias1/1 -> Sum/2
  weight1/1 -> Sum/1
  In1/1 -> weight1/1
  Sum/1 -> Out1/1

== system nn_12B/nn_2x10x10x1/Neuron Layer 1/Neuron 4/If Action Subsystem ==
  In1 : Inport
  Action Port : ActionPort  ActionPortLabel=if { }
  Sum : Sum  Inputs=|+-
  bias1 : Constant  Value=0.990025
  weight1 : Gain  Gain=0.01
  Out1 : Outport  VectorParamsAs1DForOutWhenUnconnected=off
  wires:
  bias1/1 -> Sum/2
  weight1/1 -> Sum/1
  In1/1 -> weight1/1
  Sum/1 -> Out1/1

== system nn_12B/nn_2x10x10x1/Neuron Layer 1/Neuron 4/If Action Subsystem1 ==
  In1 : Inport
  Action Port : ActionPort  ActionPortLabel=elseif { }
  Product1 : Product  RndMeth=Zero
  Sum3 : Sum  Inputs=|++
  bias4 : Constant  Value=2
  Out1 : Outport  VectorParamsAs1DForOutWhenUnconnected=off
  wires:
  In1/1 -> Product1/1, Sum3/1
  bias4/1 -> Sum3/2
  Sum3/1 -> Product1/2
  Product1/1 -> Out1/1

== system nn_12B/nn_2x10x10x1/Neuron Layer 1/Neuron 4/If Action Subsystem2 ==
  In1 : Inport
  Action Port : ActionPort  ActionPortLabel=elseif { }
  Product1 : Product  RndMeth=Zero
  Sum3 : Sum  Inputs=|-+
  bias4 : Constant  Value=2
  Out1 : Outport  VectorParamsAs1DForOutWhenUnconnected=off
  wires:
  Product1/1 -> Out1/1
  Sum3/1 -> Product1/2
  bias4/1 -> Sum3/2
  In1/1 -> Sum3/1, Product1/1

== system nn_12B/nn_2x10x10x1/Neuron Layer 1/Neuron 4/If Action Subsystem3 ==
  In1 : Inport
  Action Port : ActionPort  ActionPortLabel=else { }
  Sum : Sum  Inputs=|++
  bias1 : Constant  Value=0.990025
  weight1 : Gain  Gain=0.01
  Out1 : Outport  VectorParamsAs1DForOutWhenUnconnected=off
  wires:
  bias1/1 -> Sum/2
  weight1/1 -> Sum/1
  In1/1 -> weight1/1
  Sum/1 -> Out1/1

== system nn_12B/nn_2x10x10x1/Neuron Layer 1/Neuron 5/If Action Subsystem ==
  In1 : Inport
  Action Port : ActionPort  ActionPortLabel=if { }
  Sum : Sum  Inputs=|+-
  bias1 : Constant  Value=0.990025
  weight1 : Gain  Gain=0.01
  Out1 : Outport  VectorParamsAs1DForOutWhenUnconnected=off
  wires:
  bias1/1 -> Sum/2
  weight1/1 -> Sum/1
  In1/1 -> weight1/1
  Sum/1 -> Out1/1

== system nn_12B/nn_2x10x10x1/Neuron Layer 1/Neuron 5/If Action Subsystem1 ==
  In1 : Inport
  Action Port : ActionPort  ActionPortLabel=elseif { }
  Product1 : Product  RndMeth=Zero
  Sum3 : Sum  Inputs=|++
  bias4 : Constant  Value=2
  Out1 : Outport  VectorParamsAs1DForOutWhenUnconnected=off
  wires:
  In1/1 -> Product1/1, Sum3/1
  bias4/1 -> Sum3/2
  Sum3/1 -> Product1/2
  Product1/1 -> Out1/1

== system nn_12B/nn_2x10x10x1/Neuron Layer 1/Neuron 5/If Action Subsystem2 ==
  In1 : Inport
  Action Port : ActionPort  ActionPortLabel=elseif { }
  Product1 : Product  RndMeth=Zero
  Sum3 : Sum  Inputs=|-+
  bias4 : Constant  Value=2
  Out1 : Outport  VectorParamsAs1DForOutWhenUnconnected=off
  wires:
  Product1/1 -> Out1/1
  Sum3/1 -> Product1/2
  bias4/1 -> Sum3/2
  In1/1 -> Sum3/1, Product1/1

== system nn_12B/nn_2x10x10x1/Neuron Layer 1/Neuron 5/If Action Subsystem3 ==
  In1 : Inport
  Action Port : ActionPort  ActionPortLabel=else { }
  Sum : Sum  Inputs=|++
  bias1 : Constant  Value=0.990025
  weight1 : Gain  Gain=0.01
  Out1 : Outport  VectorParamsAs1DForOutWhenUnconnected=off
  wires:
  bias1/1 -> Sum/2
  weight1/1 -> Sum/1
  In1/1 -> weight1/1
  Sum/1 -> Out1/1

== system nn_12B/nn_2x10x10x1/Neuron Layer 1/Neuron 6/If Action Subsystem ==
  In1 : Inport
  Action Port : ActionPort  ActionPortLabel=if { }
  Sum : Sum  Inputs=|+-
  bias1 : Constant  Value=0.990025
  weight1 : Gain  Gain=0.01
  Out1 : Outport  VectorParamsAs1DForOutWhenUnconnected=off
  wires:
  Sum/1 -> Out1/1
  In1/1 -> weight1/1
  weight1/1 -> Sum/1
  bias1/1 -> Sum/2

== system nn_12B/nn_2x10x10x1/Neuron Layer 1/Neuron 6/If Action Subsystem1 ==
  In1 : Inport
  Action Port : ActionPort  ActionPortLabel=elseif { }
  Product1 : Product  RndMeth=Zero
  Sum3 : Sum  Inputs=|++
  bias4 : Constant  Value=2
  Out1 : Outport  VectorParamsAs1DForOutWhenUnconnected=off
  wires:
  Product1/1 -> Out1/1
  Sum3/1 -> Product1/2
  bias4/1 -> Sum3/2
  In1/1 -> Sum3/1, Product1/1

== system nn_12B/nn_2x10x10x1/Neuron Layer 1/Neuron 6/If Action Subsystem2 ==
  In1 : Inport
  Action Port : ActionPort  ActionPortLabel=elseif { }
  Product1 : Product  RndMeth=Zero
  Sum3 : Sum  Inputs=|-+
  bias4 : Constant  Value=2
  Out1 : Outport  VectorParamsAs1DForOutWhenUnconnected=off
  wires:
  In1/1 -> Product1/1, Sum3/1
  bias4/1 -> Sum3/2
  Sum3/1 -> Product1/2
  Product1/1 -> Out1/1

== system nn_12B/nn_2x10x10x1/Neuron Layer 1/Neuron 6/If Action Subsystem3 ==
  In1 : Inport
  Action Port : ActionPort  ActionPortLabel=else { }
  Sum : Sum  Inputs=|++
  bias1 : Constant  Value=0.990025
  weight1 : Gain  Gain=0.01
  Out1 : Outport  VectorParamsAs1DForOutWhenUnconnected=off
  wires:
  Sum/1 -> Out1/1
  In1/1 -> weight1/1
  weight1/1 -> Sum/1
  bias1/1 -> Sum/2

== system nn_12B/nn_2x10x10x1/Neuron Layer 1/Neuron 7/If Action Subsystem ==
  In1 : Inport
  Action Port : ActionPort  ActionPortLabel=if { }
  Sum : Sum  Inputs=|+-
  bias1 : Constant  Value=0.990025
  weight1 : Gain  Gain=0.01
  Out1 : Outport  VectorParamsAs1DForOutWhenUnconnected=off
  wires:
  bias1/1 -> Sum/2
  weight1/1 -> Sum/1
  In1/1 -> weight1/1
  Sum/1 -> Out1/1

== system nn_12B/nn_2x10x10x1/Neuron Layer 1/Neuron 7/If Action Subsystem1 ==
  In1 : Inport
  Action Port : ActionPort  ActionPortLabel=elseif { }
  Product1 : Product  RndMeth=Zero
  Sum3 : Sum  Inputs=|++
  bias4 : Constant  Value=2
  Out1 : Outport  VectorParamsAs1DForOutWhenUnconnected=off
  wires:
  In1/1 -> Product1/1, Sum3/1
  bias4/1 -> Sum3/2
  Sum3/1 -> Product1/2
  Product1/1 -> Out1/1

== system nn_12B/nn_2x10x10x1/Neuron Layer 1/Neuron 7/If Action Subsystem2 ==
  In1 : Inport
  Action Port : ActionPort  ActionPortLabel=elseif { }
  Product1 : Product  RndMeth=Zero
  Sum3 : Sum  Inputs=|-+
  bias4 : Constant  Value=2
  Out1 : Outport  VectorParamsAs1DForOutWhenUnconnected=off
  wires:
  Product1/1 -> Out1/1
  Sum3/1 -> Product1/2
  bias4/1 -> Sum3/2
  In1/1 -> Sum3/1, Product1/1

== system nn_12B/nn_2x10x10x1/Neuron Layer 1/Neuron 7/If Action Subsystem3 ==
  In1 : Inport
  Action Port : ActionPort  ActionPortLabel=else { }
  Sum : Sum  Inputs=|++
  bias1 : Constant  Value=0.990025
  weight1 : Gain  Gain=0.01
  Out1 : Outport  VectorParamsAs1DForOutWhenUnconnected=off
  wires:
  bias1/1 -> Sum/2
  weight1/1 -> Sum/1
  In1/1 -> weight1/1
  Sum/1 -> Out1/1

== system nn_12B/nn_2x10x10x1/Neuron Layer 1/Neuron 8/If Action Subsystem ==
  In1 : Inport
  Action Port : ActionPort  ActionPortLabel=if { }
  Sum : Sum  Inputs=|+-
  bias1 : Constant  Value=0.990025
  weight1 : Gain  Gain=0.01
  Out1 : Outport  VectorParamsAs1DForOutWhenUnconnected=off
  wires:
  bias1/1 -> Sum/2
  weight1/1 -> Sum/1
  In1/1 -> weight1/1
  Sum/1 -> Out1/1

== system nn_12B/nn_2x10x10x1/Neuron Layer 1/Neuron 8/If Action Subsystem1 ==
  In1 : Inport
  Action Port : ActionPort  ActionPortLabel=elseif { }
  Product1 : Product  RndMeth=Zero
  Sum3 : Sum  Inputs=|++
  bias4 : Constant  Value=2
  Out1 : Outport  VectorParamsAs1DForOutWhenUnconnected=off
  wires:
  In1/1 -> Product1/1, Sum3/1
  bias4/1 -> Sum3/2
  Sum3/1 -> Product1/2
  Product1/1 -> Out1/1

== system nn_12B/nn_2x10x10x1/Neuron Layer 1/Neuron 8/If Action Subsystem2 ==
  In1 : Inport
  Action Port : ActionPort  ActionPortLabel=elseif { }
  Product1 : Product  RndMeth=Zero
  Sum3 : Sum  Inputs=|-+
  bias4 : Constant  Value=2
  Out1 : Outport  VectorParamsAs1DForOutWhenUnconnected=off
  wires:
  Product1/1 -> Out1/1
  Sum3/1 -> Product1/2
  bias4/1 -> Sum3/2
  In1/1 -> Sum3/1, Product1/1

== system nn_12B/nn_2x10x10x1/Neuron Layer 1/Neuron 8/If Action Subsystem3 ==
  In1 : Inport
  Action Port : ActionPort  ActionPortLabel=else { }
  Sum : Sum  Inputs=|++
  bias1 : Constant  Value=0.990025
  weight1 : Gain  Gain=0.01
  Out1 : Outport  VectorParamsAs1DForOutWhenUnconnected=off
  wires:
  bias1/1 -> Sum/2
  weight1/1 -> Sum/1
  In1/1 -> weight1/1
  Sum/1 -> Out1/1

== system nn_12B/nn_2x10x10x1/Neuron Layer 1/Neuron 9/If Action Subsystem ==
  In1 : Inport
  Action Port : ActionPort  ActionPortLabel=if { }
  Sum : Sum  Inputs=|+-
  bias1 : Constant  Value=0.990025
  weight1 : Gain  Gain=0.01
  Out1 : Outport  VectorParamsAs1DForOutWhenUnconnected=off
  wires:
  bias1/1 -> Sum/2
  weight1/1 -> Sum/1
  In1/1 -> weight1/1
  Sum/1 -> Out1/1

== system nn_12B/nn_2x10x10x1/Neuron Layer 1/Neuron 9/If Action Subsystem1 ==
  In1 : Inport
  Action Port : ActionPort  ActionPortLabel=elseif { }
  Product1 : Product  RndMeth=Zero
  Sum3 : Sum  Inputs=|++
  bias4 : Constant  Value=2
  Out1 : Outport  VectorParamsAs1DForOutWhenUnconnected=off
  wires:
  In1/1 -> Product1/1, Sum3/1
  bias4/1 -> Sum3/2
  Sum3/1 -> Product1/2
  Product1/1 -> Out1/1

== system nn_12B/nn_2x10x10x1/Neuron Layer 1/Neuron 9/If Action Subsystem2 ==
  In1 : Inport
  Action Port : ActionPort  ActionPortLabel=elseif { }
  Product1 : Product  RndMeth=Zero
  Sum3 : Sum  Inputs=|-+
  bias4 : Constant  Value=2
  Out1 : Outport  VectorParamsAs1DForOutWhenUnconnected=off
  wires:
  Product1/1 -> Out1/1
  Sum3/1 -> Product1/2
  bias4/1 -> Sum3/2
  In1/1 -> Sum3/1, Product1/1

== system nn_12B/nn_2x10x10x1/Neuron Layer 1/Neuron 9/If Action Subsystem3 ==
  In1 : Inport
  Action Port : ActionPort  ActionPortLabel=else { }
  Sum : Sum  Inputs=|++
  bias1 : Constant  Value=0.990025
  weight1 : Gain  Gain=0.01
  Out1 : Outport  VectorParamsAs1DForOutWhenUnconnected=off
  wires:
  bias1/1 -> Sum/2
  weight1/1 -> Sum/1
  In1/1 -> weight1/1
  Sum/1 -> Out1/1

== system nn_12B/nn_2x10x10x1/Neuron Layer 2/Neuron 1/If Action Subsystem ==
  In1 : Inport
  Action Port : ActionPort  ActionPortLabel=if { }
  Sum : Sum  Inputs=|+-
  bias1 : Constant  Value=0.990025
  weight1 : Gain  Gain=0.01
  Out1 : Outport  VectorParamsAs1DForOutWhenUnconnected=off
  wires:
  bias1/1 -> Sum/2
  weight1/1 -> Sum/1
  In1/1 -> weight1/1
  Sum/1 -> Out1/1

== system nn_12B/nn_2x10x10x1/Neuron Layer 2/Neuron 1/If Action Subsystem1 ==
  In1 : Inport
  Action Port : ActionPort  ActionPortLabel=elseif { }
  Product1 : Product  RndMeth=Zero
  Sum3 : Sum  Inputs=|++
  bias4 : Constant  Value=2
  Out1 : Outport  VectorParamsAs1DForOutWhenUnconnected=off
  wires:
  In1/1 -> Product1/1, Sum3/1
  bias4/1 -> Sum3/2
  Sum3/1 -> Product1/2
  Product1/1 -> Out1/1

== system nn_12B/nn_2x10x10x1/Neuron Layer 2/Neuron 1/If Action Subsystem2 ==
  In1 : Inport
  Action Port : ActionPort  ActionPortLabel=elseif { }
  Product1 : Product  RndMeth=Zero
  Sum3 : Sum  Inputs=|-+
  bias4 : Constant  Value=2
  Out1 : Outport  VectorParamsAs1DForOutWhenUnconnected=off
  wires:
  Product1/1 -> Out1/1
  Sum3/1 -> Product1/2
  bias4/1 -> Sum3/2
  In1/1 -> Sum3/1, Product1/1

== system nn_12B/nn_2x10x10x1/Neuron Layer 2/Neuron 1/If Action Subsystem3 ==
  In1 : Inport
  Action Port : ActionPort  ActionPortLabel=else { }
  Sum : Sum  Inputs=|++
  bias1 : Constant  Value=0.990025
  weight1 : Gain  Gain=0.01
  Out1 : Outport  VectorParamsAs1DForOutWhenUnconnected=off
  wires:
  bias1/1 -> Sum/2
  weight1/1 -> Sum/1
  In1/1 -> weight1/1
  Sum/1 -> Out1/1

== system nn_12B/nn_2x10x10x1/Neuron Layer 2/Neuron 10/If Action Subsystem ==
  In1 : Inport
  Action Port : ActionPort  ActionPortLabel=if { }
  Sum : Sum  Inputs=|+-
  bias1 : Constant  Value=0.990025
  weight1 : Gain  Gain=0.01
  Out1 : Outport  VectorParamsAs1DForOutWhenUnconnected=off
  wires:
  Sum/1 -> Out1/1
  In1/1 -> weight1/1
  weight1/1 -> Sum/1
  bias1/1 -> Sum/2

== system nn_12B/nn_2x10x10x1/Neuron Layer 2/Neuron 10/If Action Subsystem1 ==
  In1 : Inport
  Action Port : ActionPort  ActionPortLabel=elseif { }
  Product1 : Product  RndMeth=Zero
  Sum3 : Sum  Inputs=|++
  bias4 : Constant  Value=2
  Out1 : Outport  VectorParamsAs1DForOutWhenUnconnected=off
  wires:
  Product1/1 -> Out1/1
  Sum3/1 -> Product1/2
  bias4/1 -> Sum3/2
  In1/1 -> Sum3/1, Product1/1

== system nn_12B/nn_2x10x10x1/Neuron Layer 2/Neuron 10/If Action Subsystem2 ==
  In1 : Inport
  Action Port : ActionPort  ActionPortLabel=elseif { }
  Product1 : Product  RndMeth=Zero
  Sum3 : Sum  Inputs=|-+
  bias4 : Constant  Value=2
  Out1 : Outport  VectorParamsAs1DForOutWhenUnconnected=off
  wires:
  In1/1 -> Product1/1, Sum3/1
  bias4/1 -> Sum3/2
  Sum3/1 -> Product1/2
  Product1/1 -> Out1/1

== system nn_12B/nn_2x10x10x1/Neuron Layer 2/Neuron 10/If Action Subsystem3 ==
  In1 : Inport
  Action Port : ActionPort  ActionPortLabel=else { }
  Sum : Sum  Inputs=|++
  bias1 : Constant  Value=0.990025
  weight1 : Gain  Gain=0.01
  Out1 : Outport  VectorParamsAs1DForOutWhenUnconnected=off
  wires:
  Sum/1 -> Out1/1
  In1/1 -> weight1/1
  weight1/1 -> Sum/1
  bias1/1 -> Sum/2

== system nn_12B/nn_2x10x10x1/Neuron Layer 2/Neuron 2/If Action Subsystem ==
  In1 : Inport
  Action Port : ActionPort  ActionPortLabel=if { }
  Sum : Sum  Inputs=|+-
  bias1 : Constant  Value=0.990025
  weight1 : Gain  Gain=0.01
  Out1 : Outport  VectorParamsAs1DForOutWhenUnconnected=off
  wires:
  Sum/1 -> Out1/1
  In1/1 -> weight1/1
  weight1/1 -> Sum/1
  bias1/1 -> Sum/2

== system nn_12B/nn_2x10x10x1/Neuron Layer 2/Neuron 2/If Action Subsystem1 ==
  In1 : Inport
  Action Port : ActionPort  ActionPortLabel=elseif { }
  Product1 : Product  RndMeth=Zero
  Sum3 : Sum  Inputs=|++
  bias4 : Constant  Value=2
  Out1 : Outport  VectorParamsAs1DForOutWhenUnconnected=off
  wires:
  Product1/1 -> Out1/1
  Sum3/1 -> Product1/2
  bias4/1 -> Sum3/2
  In1/1 -> Sum3/1, Product1/1

== system nn_12B/nn_2x10x10x1/Neuron Layer 2/Neuron 2/If Action Subsystem2 ==
  In1 : Inport
  Action Port : ActionPort  ActionPortLabel=elseif { }
  Product1 : Product  RndMeth=Zero
  Sum3 : Sum  Inputs=|-+
  bias4 : Constant  Value=2
  Out1 : Outport  VectorParamsAs1DForOutWhenUnconnected=off
  wires:
  In1/1 -> Product1/1, Sum3/1
  bias4/1 -> Sum3/2
  Sum3/1 -> Product1/2
  Product1/1 -> Out1/1

== system nn_12B/nn_2x10x10x1/Neuron Layer 2/Neuron 2/If Action Subsystem3 ==
  In1 : Inport
  Action Port : ActionPort  ActionPortLabel=else { }
  Sum : Sum  Inputs=|++
  bias1 : Constant  Value=0.990025
  weight1 : Gain  Gain=0.01
  Out1 : Outport  VectorParamsAs1DForOutWhenUnconnected=off
  wires:
  Sum/1 -> Out1/1
  In1/1 -> weight1/1
  weight1/1 -> Sum/1
  bias1/1 -> Sum/2

== system nn_12B/nn_2x10x10x1/Neuron Layer 2/Neuron 3/If Action Subsystem ==
  In1 : Inport
  Action Port : ActionPort  ActionPortLabel=if { }
  Sum : Sum  Inputs=|+-
  bias1 : Constant  Value=0.990025
  weight1 : Gain  Gain=0.01
  Out1 : Outport  VectorParamsAs1DForOutWhenUnconnected=off
  wires:
  bias1/1 -> Sum/2
  weight1/1 -> Sum/1
  In1/1 -> weight1/1
  Sum/1 -> Out1/1

== system nn_12B/nn_2x10x10x1/Neuron Layer 2/Neuron 3/If Action Subsystem1 ==
  In1 : Inport
  Action Port : ActionPort  ActionPortLabel=elseif { }
  Product1 : Product  RndMeth=Zero
  Sum3 : Sum  Inputs=|++
  bias4 : Constant  Value=2
  Out1 : Outport  VectorParamsAs1DForOutWhenUnconnected=off
  wires:
  In1/1 -> Product1/1, Sum3/1
  bias4/1 -> Sum3/2
  Sum3/1 -> Product1/2
  Product1/1 -> Out1/1

== system nn_12B/nn_2x10x10x1/Neuron Layer 2/Neuron 3/If Action Subsystem2 ==
  In1 : Inport
  Action Port : ActionPort  ActionPortLabel=elseif { }
  Product1 : Product  RndMeth=Zero
  Sum3 : Sum  Inputs=|-+
  bias4 : Constant  Value=2
  Out1 : Outport  VectorParamsAs1DForOutWhenUnconnected=off
  wires:
  Product1/1 -> Out1/1
  Sum3/1 -> Product1/2
  bias4/1 -> Sum3/2
  In1/1 -> Sum3/1, Product1/1

== system nn_12B/nn_2x10x10x1/Neuron Layer 2/Neuron 3/If Action Subsystem3 ==
  In1 : Inport
  Action Port : ActionPort  ActionPortLabel=else { }
  Sum : Sum  Inputs=|++
  bias1 : Constant  Value=0.990025
  weight1 : Gain  Gain=0.01
  Out1 : Outport  VectorParamsAs1DForOutWhenUnconnected=off
  wires:
  bias1/1 -> Sum/2
  weight1/1 -> Sum/1
  In1/1 -> weight1/1
  Sum/1 -> Out1/1

== system nn_12B/nn_2x10x10x1/Neuron Layer 2/Neuron 4/If Action Subsystem ==
  In1 : Inport
  Action Port : ActionPort  ActionPortLabel=if { }
  Sum : Sum  Inputs=|+-
  bias1 : Constant  Value=0.990025
  weight1 : Gain  Gain=0.01
  Out1 : Outport  VectorParamsAs1DForOutWhenUnconnected=off
  wires:
  bias1/1 -> Sum/2
  weight1/1 -> Sum/1
  In1/1 -> weight1/1
  Sum/1 -> Out1/1

== system nn_12B/nn_2x10x10x1/Neuron Layer 2/Neuron 4/If Action Subsystem1 ==
  In1 : Inport
  Action Port : ActionPort  ActionPortLabel=elseif { }
  Product1 : Product  RndMeth=Zero
  Sum3 : Sum  Inputs=|++
  bias4 : Constant  Value=2
  Out1 : Outport  VectorParamsAs1DForOutWhenUnconnected=off
  wires:
  In1/1 -> Product1/1, Sum3/1
  bias4/1 -> Sum3/2
  Sum3/1 -> Product1/2
  Product1/1 -> Out1/1

== system nn_12B/nn_2x10x10x1/Neuron Layer 2/Neuron 4/If Action Subsystem2 ==
  In1 : Inport
  Action Port : ActionPort  ActionPortLabel=elseif { }
  Product1 : Product  RndMeth=Zero
  Sum3 : Sum  Inputs=|-+
  bias4 : Constant  Value=2
  Out1 : Outport  VectorParamsAs1DForOutWhenUnconnected=off
  wires:
  Product1/1 -> Out1/1
  Sum3/1 -> Product1/2
  bias4/1 -> Sum3/2
  In1/1 -> Sum3/1, Product1/1

== system nn_12B/nn_2x10x10x1/Neuron Layer 2/Neuron 4/If Action Subsystem3 ==
  In1 : Inport
  Action Port : ActionPort  ActionPortLabel=else { }
  Sum : Sum  Inputs=|++
  bias1 : Constant  Value=0.990025
  weight1 : Gain  Gain=0.01
  Out1 : Outport  VectorParamsAs1DForOutWhenUnconnected=off
  wires:
  bias1/1 -> Sum/2
  weight1/1 -> Sum/1
  In1/1 -> weight1/1
  Sum/1 -> Out1/1

== system nn_12B/nn_2x10x10x1/Neuron Layer 2/Neuron 5/If Action Subsystem ==
  In1 : Inport
  Action Port : ActionPort  ActionPortLabel=if { }
  Sum : Sum  Inputs=|+-
  bias1 : Constant  Value=0.990025
  weight1 : Gain  Gain=0.01
  Out1 : Outport  VectorParamsAs1DForOutWhenUnconnected=off
  wires:
  bias1/1 -> Sum/2
  weight1/1 -> Sum/1
  In1/1 -> weight1/1
  Sum/1 -> Out1/1

== system nn_12B/nn_2x10x10x1/Neuron Layer 2/Neuron 5/If Action Subsystem1 ==
  In1 : Inport
  Action Port : ActionPort  ActionPortLabel=elseif { }
  Product1 : Product  RndMeth=Zero
  Sum3 : Sum  Inputs=|++
  bias4 : Constant  Value=2
  Out1 : Outport  VectorParamsAs1DForOutWhenUnconnected=off
  wires:
  In1/1 -> Product1/1, Sum3/1
  bias4/1 -> Sum3/2
  Sum3/1 -> Product1/2
  Product1/1 -> Out1/1

== system nn_12B/nn_2x10x10x1/Neuron Layer 2/Neuron 5/If Action Subsystem2 ==
  In1 : Inport
  Action Port : ActionPort  ActionPortLabel=elseif { }
  Product1 : Product  RndMeth=Zero
  Sum3 : Sum  Inputs=|-+
  bias4 : Constant  Value=2
  Out1 : Outport  VectorParamsAs1DForOutWhenUnconnected=off
  wires:
  Product1/1 -> Out1/1
  Sum3/1 -> Product1/2
  bias4/1 -> Sum3/2
  In1/1 -> Sum3/1, Product1/1
